simulink subsystem "Guidance"  (R2026a)
settings: Solver=VariableStepAuto
values from neighbouring files (symbols this model uses):
  guidanceParams = 0.0    [controllerParams.sldd]
settings Model: DataDictionary=controllerParams.sldd  EnableAccessToBaseWorkspace=off  Creator=maxhu  LastModifiedBy=maxhu

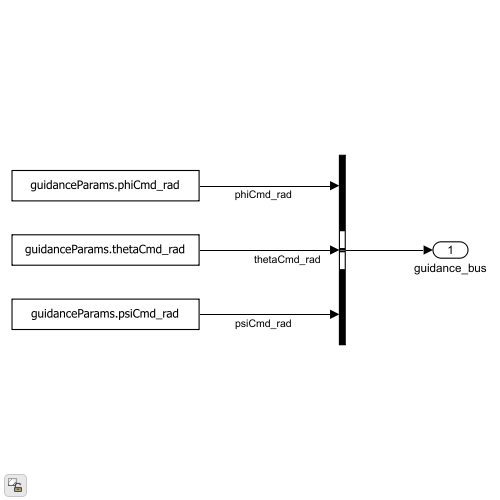
[thumbnail: Simulink's stored preview of the top-level diagram]
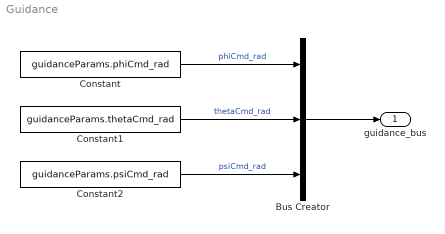
== system Guidance ==
  Bus Creator : BusCreator  Inputs=3
  Constant : Constant  Value=guidanceParams.phiCmd_rad
  Constant1 : Constant  Value=guidanceParams.thetaCmd_rad
  Constant2 : Constant  Value=guidanceParams.psiCmd_rad
  guidance_bus : Outport
  wires:
  Bus Creator/1 -> guidance_bus/1
  Constant/1 -> Bus Creator/1  "phiCmd_rad"
  Constant2/1 -> Bus Creator/3  "psiCmd_rad"
  Constant1/1 -> Bus Creator/2  "thetaCmd_rad"
